simulink model "InTube_HT_Check_Rside"  (R2025a)
settings: Solver=VariableStepAuto  StartTime=0.0  StopTime=10.0  RelTol=1e-3
undefined symbols (not defined in the file): GeoCondition, mdot_in
libraries: fl_lib x19, nesl_utility x2, simulink x1, SimscapeFluids_lib x1
settings Model: Creator=20112  LastModifiedBy=20112

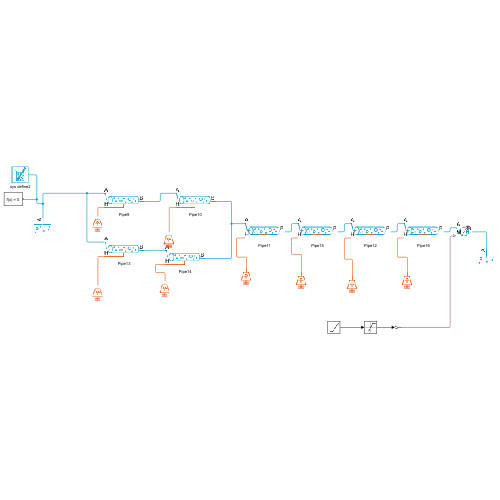
[thumbnail: Simulink's stored preview of the top-level diagram]
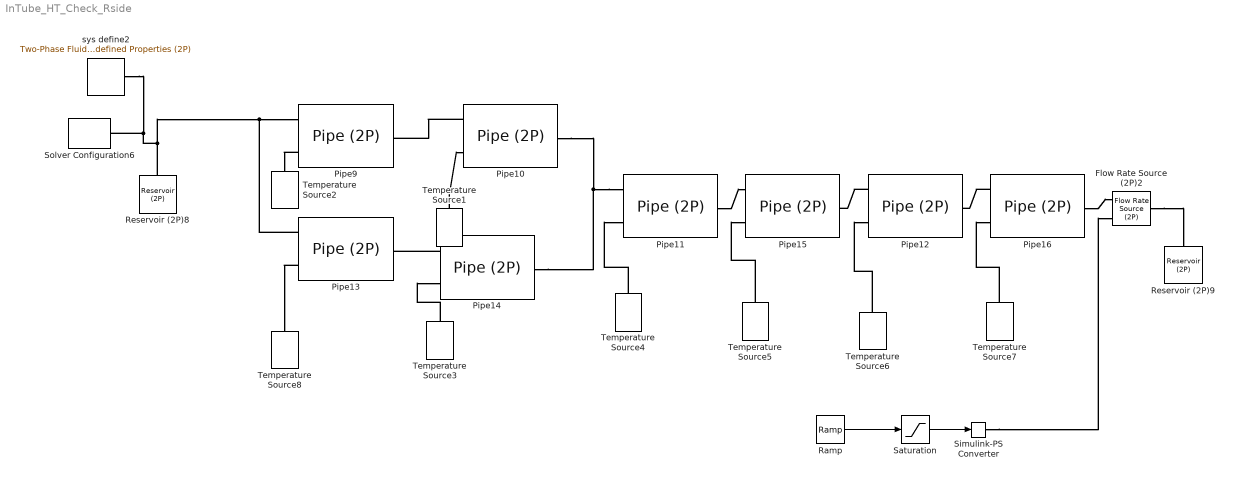
== system InTube_HT_Check_Rside ==
  Flow Rate Source (2P)2 : fl_lib/Two-Phase Fluid/Sources/Flow Rate Source (2P)  source_type=foundation.enum.constant_controlled.controlled  flow_type=foundation.enum.mass_volumetric_flow.mass  mass_flow=20e-3 kg/s  volumetric_flow=0 m^3/s  power_spec=foundation.enum.power_spec.none  area_A=pi*(GeoCondition.D)^2/4 m^2  area_B=pi*(GeoCondition.D)^2/4 m^2
      settings: InternalSimscapePortConfiguration="{\"Bottom\":[],\"Left\":[{\"id\":\"A\",\"label\":\"A\",\"type\":\"foundation.two_phase_fluid.two_phase_fluid\"},{\"id\":\"M\",\"label\":\"M\",\"type\":\"input\"}],\"Right\":[{\"id\":\"B\",\"label\":\"B\",\"type\":\"foundation.two_phase_fluid.two_phase_fluid\"}],\"Top\":[]}"
  Pipe{9..16} (8 alike) : fl_lib/Two-Phase Fluid/Elements/Pipe (2P)  length=GeoCondition.L m  area=pi*(GeoCondition.D)^2/4 m^2  Dh=GeoCondition.D m  length_add=0 m  roughness=GeoCondition.r m  Re_lam=2000  Re_tur=4000  shape_factor=64  Nu_lam=3.66  inertia=false  energy_spec=foundation.enum.energy_spec.enthalpy  p_init=1 MPa  T_init=310 K  x_init=0.5  alpha_init=0.5  h_init=300 kJ/kg  u_init=264.74 kJ/kg  mdot_init=0 kg/s  time_constant=0.1 s
      settings: InternalSimscapePortConfiguration="{\"Bottom\":[],\"Left\":[{\"id\":\"A\",\"label\":\"A\",\"type\":\"foundation.two_phase_fluid.two_phase_fluid\"},{\"id\":\"H\",\"label\":\"H\",\"type\":\"foundation.thermal.thermal\"}],\"Right\":[{\"id\":\"B\",\"label\":\"B\",\"type\":\"foundation.two_phase_fluid.two_phase_fluid\"}],\"Top\":[]}"
  Ramp : simulink/Sources/Ramp  slope=1e-3  start=0  InitialOutput=0
  Reservoir (2P)8 : fl_lib/Two-Phase Fluid/Elements/Reservoir (2P)  pressure_spec=foundation.enum.ReservoirPressureSpec2P.Specified  reservoir_pressure=p_in MPa  reservoir_condensing_temperature=373.15 K  reservoir_evaporating_temperature=373.15 K  energy_spec=foundation.enum.ReservoirEnergySpec2P.Enthalpy  reservoir_temperature=310 K  reservoir_quality=0.5  reservoir_void_fraction=0.5  reservoir_enthalpy=h_inlet kJ/kg  reservoir_internal_energy=264.74 kJ/kg  reservoir_subcooling=5 deltaK  reservoir_superheating=5 deltaK  area_A=pi*(GeoCondition.D)^2/4 m^2
  Reservoir (2P)9 : fl_lib/Two-Phase Fluid/Elements/Reservoir (2P)  pressure_spec=foundation.enum.ReservoirPressureSpec2P.Specified  reservoir_pressure=0.95 MPa  reservoir_condensing_temperature=373.15 K  reservoir_evaporating_temperature=373.15 K  energy_spec=foundation.enum.ReservoirEnergySpec2P.Enthalpy  reservoir_temperature=310 K  reservoir_quality=0.5  reservoir_void_fraction=0.5  reservoir_enthalpy=300 kJ/kg  reservoir_internal_energy=1500 kJ/kg  reservoir_subcooling=5 deltaK  reservoir_superheating=5 deltaK  area_A=pi*(GeoCondition.D)^2/4 m^2
  Saturation : Saturate  UpperLimit=mdot_in  LowerLimit=0
  Simulink-PS Converter : nesl_utility/Simulink-PS Converter  PhysicalDomain=network_engine_domain  SubClassName=ps_input  LeftPortType=input  RightPortType=output  PseudoPeriodic=off  Frequencies=[]  NoiseDistribution=none  NoiseParameters=[]  Unit=kg/s  AffineConversion=on  FilteringAndDerivatives=provide  SimscapeFilterOrder=1  InputFilterTimeConstant=0.001  UdotUserProvided=0
  Solver Configuration6 : nesl_utility/Solver Configuration  PhysicalDomain=network_engine_domain  SubClassName=solver  LeftPortType=input  RightPortType=generic  Tones=[]  Harmonics=[]  SimulateNoise=off  Profile=off  UseLocalSampling=off  EnableSwitchedLinearOptims=on  FrequencyDomain=off  UseCCode=off  RelTol=0.001  AbsTol=0.001  MinStep=1e-09  ToWorkspace=off  RevertToSquareIcSolve=off  NumHomotopyIterations=100  PhasorMode=off  PhasorModeNumHarmonics=1  ConsistencySolver=NEWTON_XTOL_AFTER_FTOL  IndexReductionMethod=DerivativeReplacement  DoDC=off  ResidualTolerance=1e-09  ConsistencyTolSource=GLOBAL  ConsistencyAbsTol=0.001  ConsistencyRelTol=0.001  ConsistencyTolFactor=0.001  UseLocalSolver=off  LocalSolverChoice=NE_BACKWARD_EULER_ADVANCER  ResolveIndetEquations=on  FunctionEvalNumThread=1  LocalSolverSampleTime=0.001  DoFixedCost=off  MaxNonlinIter=3  MaxModeIter=2  ComputeImpulses=off  ImpulseIterations=2  LinearAlgebra=auto  LinearAlgebraNumThread=0  EquationFormulation=NE_TIME_EF  DelaysMemoryBudget=1024  AutomaticFiltering=on  FilteringTimeConstant=0.001  PartitionStorageMethod=AS_NEEDED  PartitionMemoryBudget=1024  PartitionMethod=ROBUST  MultibodyUseLocalSolver=off  MultibodyLocalSolverChoice=ODE1  MultibodyLocalSolverSampleTime=0.001
  Temperature Source{1..8} (8 alike) : fl_lib/Thermal/Thermal Sources/Temperature Source  temperature=T_wall K
  sys define2 : SimscapeFluids_lib/Two-Phase Fluid/Utilities/Two-Phase Fluid Predefined Properties (2P)  fluid=fluids.two_phase_fluid.utilities.enum.Fluid.R134a  p_atm=0.101325 MPa  properties_range_check=simscape.enum.assert.action.error  q_rev=0.01 Pa
  wires:
  Ramp/1 -> Saturation/1
  Saturation/1 -> Simulink-PS Converter/1
  connections:
  Pipe13/LConn1 -- Reservoir (2P)8/LConn1 -- sys define2/RConn1 -- Solver Configuration6/RConn1 -- Pipe9/LConn1
  Pipe11/LConn1 -- Pipe10/RConn1 -- Pipe14/RConn1
  Pipe9/LConn2 -- Temperature Source2/LConn1
  Temperature Source5/LConn1 -- Pipe15/LConn2
  Pipe14/LConn1 -- Pipe13/RConn1
  Pipe16/LConn1 -- Pipe12/RConn1
  Temperature Source6/LConn1 -- Pipe12/LConn2
  Pipe10/LConn1 -- Pipe9/RConn1
  Temperature Source4/LConn1 -- Pipe11/LConn2
  Temperature Source1/LConn1 -- Pipe10/LConn2
  Simulink-PS Converter/RConn1 -- Flow Rate Source (2P)2/LConn2
  Flow Rate Source (2P)2/RConn1 -- Reservoir (2P)9/LConn1
  Temperature Source3/LConn1 -- Pipe14/LConn2
  Pipe13/LConn2 -- Temperature Source8/LConn1
  Pipe12/LConn1 -- Pipe15/RConn1
  Pipe16/RConn1 -- Flow Rate Source (2P)2/LConn1
  Pipe11/RConn1 -- Pipe15/LConn1
  Temperature Source7/LConn1 -- Pipe16/LConn2
